simulink model "sl_subsys_while2"  (Simulink 6.0)
settings: Solver=FixedStepDiscrete  StartTime=0.0  StopTime=1  FixedStep=1  RelTol=1e-3
settings Model: CovMetricSettings=d  Creator=The MathWorks Inc.  LastModifiedBy=batserve  ExtModeAutoUpdateStatusClock=off
settings OptimizationCC: BooleanDataType=off
settings DebuggingCC: CheckExecutionContextPreStartOutputMsg=on  CheckExecutionContextRuntimeOutputMsg=on  SolverPrmCheckMsg=none
settings HardwareCC: TargetUnknown=on

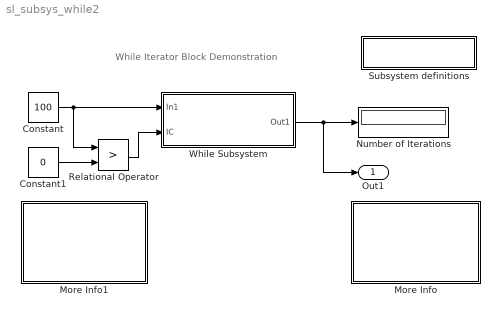
== system sl_subsys_while2 ==
  note: While Iterator Block Demonstration
  " Subsystem definitions" : Subsystem  PropExecContextAcrossSSBoundary=on
      settings: OpenFcn=helpview([matlabroot,'/toolbox/simulink/simdemos/sl_subsys_definitions.html']);
      mask Display: disp('Subsystem\ndefinitions')
  Constant : Constant  Value=100
  Constant1 : Constant  Value=0
  More Info : Subsystem  PropExecContextAcrossSSBoundary=on
      mask Display: disp('Double click\nhere for\ninformation on\nthis demonstration')
  More Info1 : Subsystem  PropExecContextAcrossSSBoundary=on
      settings: OpenFcn=simcad(bdroot);
      mask Display: disp('Double click\nhere for\nSimulink Help')
  Number of Iterations : Display
  Relational Operator : RelationalOperator  Operator=>  InputSameDT=on
  While Subsystem : Subsystem  TreatAsAtomicUnit=on  PropExecContextAcrossSSBoundary=on
  Out1 : Outport
  wires:
  Constant/1 -> While Subsystem/1(In1), Relational Operator/1
  While Subsystem/1(Out1) -> Number of Iterations/1, Out1/1
  Relational Operator/1 -> While Subsystem/2(IC)
  Constant1/1 -> Relational Operator/2

== system sl_subsys_while2/ Subsystem definitions ==

== system sl_subsys_while2/More Info ==
  note: While Iterator Block Demonstration
  note: This model demonstrates how a While Iterator block can be used to run the blocks in
      | a subsystem multiple number of times.  In this case, there is a counter in the While
      | Subsystem that adds up the numbers from 1 to N, where N is the number of iterations
      | that have been run.  The counter runs while this value is less than the input value to
      | the subsystem.  The number of iterations it took to exceed this value is shown in the
      | display.  In order to avoid an infinite loop, we have set the maximum number of iterations
      | in the do-while loop to be 1000.  This can be seen by double-clicking the While Iterator
      | block.   Also, since the algorithm does not make sense for non-positive inputs, we do
      | not run any of the blocks in the While Subsystem if the input is less than one.

== system sl_subsys_while2/More Info1 ==

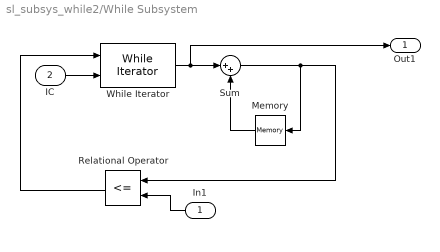
== system sl_subsys_while2/While Subsystem ==
  In1 : Inport  Orientation=left  Port=1  LatchInput=off
  IC : Inport  Port=2  LatchInput=off
  Memory : Memory  Orientation=left  InheritSampleTime=on
  Relational Operator : RelationalOperator  Orientation=left  Operator=<=  InputSameDT=on
  Sum : Sum  Inputs=|++  SaturateOnIntegerOverflow=on  InputSameDT=on
  While Iterator : WhileIterator  MaxIters=1000  ResetStates=reset  ShowIterationPort=on  OutputDataType=double
  Out1 : Outport
  wires:
  In1/1 -> Relational Operator/2
  Relational Operator/1 -> While Iterator/1
  While Iterator/1 -> Sum/1, Out1/1
  Sum/1 -> Relational Operator/1, Memory/1
  Memory/1 -> Sum/2
  IC/1 -> While Iterator/2
